simulink model "BANSHEE_GOTO"  (Simulink 8.1)
settings: Solver=ode1  StartTime=0.0  StopTime=inf  FixedStep=Ts  MaxStep=1e-3  RelTol=1e-3
PostLoadFcn:
  | BANSHEE_init;
InitFcn:
  | BANSHEE_init;
values from neighbouring files (symbols this model uses):
  F1 = xlsread('F1_relay_banshee.xlsx')    [relay_settings_init.m]
  F2 = xlsread('F2_relay_banshee.xlsx')    [relay_settings_init.m]
  F3 = xlsread('F3_relay_banshee.xlsx')    [relay_settings_init.m]
  Ts = 100E-6    (= 0.0001)    [BANSHEE_init.m]
undefined symbols (not defined in the file or in its folder): cable_spec, fdesignblkfcn, Feeder1_lib, Feeder2_lib, Feeder3_lib, gcbh, generic_ethernet_cb, Left, relay_housing_lib, SM_UtilityService, SS_F1_RELAY_HOUSING, SS_F2_RELAY_HOUSING, SS_F3_RELAY_HOUSING, SS_Feeder1, SS_Feeder2, SS_Feeder3, type, utility_service_lib, V
libraries: breaker_lib x51, rtio_generic_modbus x43, relay_modbus_lib x42, cables_lib x34, artemis x24, transformer_lib x24, Load_lib x18, simulink x16, ssn_lib x16, rtlab x15, rtio_opalrt_common x15, PQFV_lib x8
(part 2 of 5)

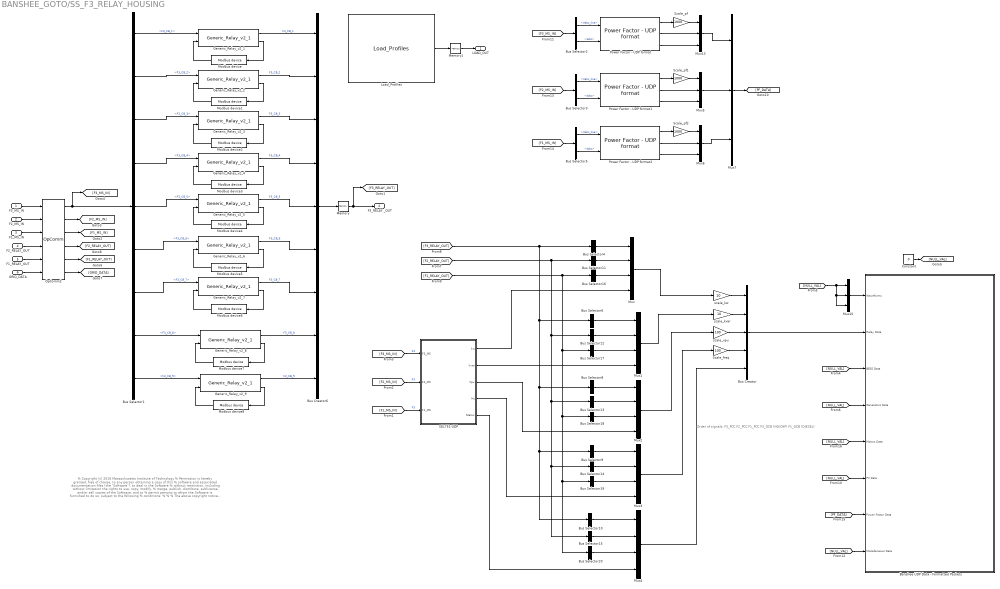
== system BANSHEE_GOTO/SS_F3_RELAY_HOUSING ==
  note: % Copyright (c) 2016 Massachusetts Institute of Technology
      | % Permission is hereby granted, free of charge, to any person obtaining a copy of this
      | % software and associated documentation files (the "Software"), to deal in the Software
      | % without restriction, including without limitation the rights to use, copy, modify,
      | % merge, publish, distribute, sublicense, and/or sell copies of the Software, and to
      | % permit persons to whom the Software is furnished to do so, subject to the following
      | % conditions:
      | %
      | %
      | % The above copyright notice and this permission notice shall be included in
      | % all copies or substantial portions of the Software.
      | %
      | % THE SOFTWARE IS PROVIDED "AS IS", WITHOUT WARRANTY OF ANY KIND, EXPRESS OR IMPLIED,
      | % INCLUDING BUT NOT LIMITED TO THE WARRANTIES OF MERCHANTABILITY, FITNESS FOR A
      | % PARTICULAR PURPOSE AND NONINFRINGEMENT. IN NO EVENT SHALL THE AUTHORS OR COPYRIGHT
      | % HOLDERS BE LIABLE FOR ANY CLAIM, DAMAGES OR OTHER LIABILITY, WHETHER IN AN ACTION
      | % OF CONTRACT, TORT OR OTHERWISE, ARISING FROM, OUT OF OR IN CONNECTION WITH THE
      | % SOFTWARE OR THE USE OR OTHER DEALINGS IN THE SOFTWARE.
      | %
      | %
      | %%
  note: Order of signals:
      | F3_PCC
      | F2_PCC
      | F1_PCC
      | F3_GCB (NG/CHP)
      | F1_GCB (DIESEL)
  F3_MS_IN : Inport
  F2_MS_IN : Inport  Port=2
  F1_MS_IN : Inport  Port=3
  F2_RELAY_OUT : Inport  Port=4
  F1_RELAY_OUT : Inport  Port=5
  GRID_DATA : Inport  Port=6
  Banshee UDP Data - Formatted Packets : Subsystem  mask(UDP Data Block){ProfileID=2, NumOfWaveforms=[0, 0, 0], NumOfRelays=[47, [10, 10, 100, 100]], NumOfBatteries=0, NumOfGensets=0, NumOfMotors=0, NumOfPVs=0, NumOfPF=[3, [1000, 1000, 1000]], NumOfMiscellaneousDataScales=0, NumOfMiscellaneousDataSignalsScales=0}
      mask prompts: ProfileID "Profile ID"; NumOfWaveforms "Waveform Data"; NumOfRelays "Relay Data"; NumOfBatteries "# of Batteries"; NumOfGensets "# of Gensets"; NumOfMotors "# of Motors"; NumOfPVs "# of PVs"; NumOfPF "Power Factor Data"; NumOfMiscellaneousDataScales "Misc. Data - No. of Scale Factors"; NumOfMiscellaneousDataSignalsScales "Misc. - No. Signals and Scale Values"
      mask help:
      | * All signal scaling should be external to this block
      |
      | Profile ID: (1-Sheriff, 2-Banshee, 3-Canary, 4-Siren)
      |
      | Waveforms Data: No. of per phase waveforms sent at 5Hz rate, point per waveforms [dt=80us, 208; dt=100us, 166], and scaling factor.
      | -Input format: [No. of waveforms, No. of datapoints, scale]
      | -Ex. for Canary:[3, 166, 100]
      |
      | Relay Data: No. of relays feeding packet data to breakers in display - mapped/indexed in ascending order
      | -Packet order: Active power(kW), reactive power(kVAR), voltage(per-unit), frequency (Hz), breaker status (1:closed, 0:open)
      | -Input format: [No. of Relays, [scale_kW, scale_kVAR, scale_Vpu, scale_Hz]]
      | -Ex. for Canary:[4, [10, 10, 100, 100]]
      |
      | No. of Batteries: TBD
      | -Ex. for Canary: [0]
      | No. of Generators: TBD
      | -Ex. for Canary: [0]
      |
      | Motors Data: No. of motors monitored in the system. Currently, only looking at motor on/off state.
      | -Input format: [No. of motors]
      | -Ex. for Canary: [1]
      |
      | No. of PV: TBD
      | -Ex. for Canary: [0]
      |
      | Power Factor Data: No. of power factors to be displayed in the system, and corresponding scale values.
      | -Packet order: power factor, import/export, lagging/leading
      | -Input format: [No. of Power Factors, [scale_pf]]
      | -Ex. for Canary:[1, [1000]]
      |
      | Misc. Data - No. of Scale factor: NUmber of scale factors to be applied to each signal-set.
      | -Ex. for Canary: [3]
      |
      | Misc. Data - No. of Signals and Scale Values: Size of signal set and scale value to be applied to the signal-set.
      | -Ex. for Canary: [[1, 1000], [6, 100], [3, 10]]
  Bus Creator : BusCreator  Inputs=5
  Bus Creator6 : BusCreator  Inputs=9
  Bus Selector1 : BusSelector  OutputSignals=CB_DATA.F3_CB_1,CB_DATA.F3_CB_2,CB_DATA.F3_CB_3,CB_DATA.F3_CB_4,CB_DATA.F3_CB_5,CB_DATA.F3_CB_6,CB_DATA.F3_CB_7,CB_DATA.F3_CB_8,CB_DATA.F3_CB_9
  Bus Selector10 : BusSelector  OutputSignals=F3_CB_1.m.status,F3_CB_2.m.status,F3_CB_3.m.status,F3_CB_4.m.status,F3_CB_5.m.status,F3_CB_6.m.status,F3_CB_7.m.status,F3_CB_8.m.status,F3_CB_9.m.status  OutputAsBus=on
  Bus Selector11 : BusSelector  OutputSignals=F2_CB_1.m.kw,F2_CB_2.m.kw,F2_CB_3.m.kw,F2_CB_4.m.kw,F2_CB_5.m.kw,F2_CB_6.m.kw,F2_CB_7.m.kw,F2_CB_8.m.kw,F2_CB_9.m.kw,F2_CB_10.m.kw,F2_CB_11.m.kw,F2_CB_12.m.kw,F2_CB_13.m.kw,F2_CB_14.m.kw,F2_CB_15.m.kw,F2_CB_16.m.kw,F2_CB_17.m.kw,F2_CB_18.m.kw,F2_CB_19.m.kw  OutputAsBus=on
  Bus Selector12 : BusSelector  OutputSignals=F2_CB_1.m.kvar,F2_CB_2.m.kvar,F2_CB_3.m.kvar,F2_CB_4.m.kvar,F2_CB_5.m.kvar,F2_CB_6.m.kvar,F2_CB_7.m.kvar,F2_CB_8.m.kvar,F2_CB_9.m.kvar,F2_CB_10.m.kvar,F2_CB_11.m.kvar,F2_CB_12.m.kvar,F2_CB_13.m.kvar,F2_CB_14.m.kvar,F2_CB_15.m.kvar,F2_CB_16.m.kvar,F2_CB_17.m.kvar,F2_CB_18.m.kvar,F2_CB_19.m.kvar  OutputAsBus=on
  Bus Selector13 : BusSelector  OutputSignals=F2_CB_1.m.Vpu,F2_CB_2.m.Vpu,F2_CB_3.m.Vpu,F2_CB_4.m.Vpu,F2_CB_5.m.Vpu,F2_CB_6.m.Vpu,F2_CB_7.m.Vpu,F2_CB_8.m.Vpu,F2_CB_9.m.Vpu,F2_CB_10.m.Vpu,F2_CB_11.m.Vpu,F2_CB_12.m.Vpu,F2_CB_13.m.Vpu,F2_CB_14.m.Vpu,F2_CB_15.m.Vpu,F2_CB_16.m.Vpu,F2_CB_17.m.Vpu,F2_CB_18.m.Vpu,F2_CB_19.m.Vpu  OutputAsBus=on
  Bus Selector14 : BusSelector  OutputSignals=F2_CB_1.m.Hz,F2_CB_2.m.Hz,F2_CB_3.m.Hz,F2_CB_4.m.Hz,F2_CB_5.m.Hz,F2_CB_6.m.Hz,F2_CB_7.m.Hz,F2_CB_8.m.Hz,F2_CB_9.m.Hz,F2_CB_10.m.Hz,F2_CB_11.m.Hz,F2_CB_12.m.Hz,F2_CB_13.m.Hz,F2_CB_14.m.Hz,F2_CB_15.m.Hz,F2_CB_16.m.Hz,F2_CB_17.m.Hz,F2_CB_18.m.Hz,F2_CB_19.m.Hz  OutputAsBus=on
  Bus Selector15 : BusSelector  OutputSignals=F2_CB_1.m.status,F2_CB_2.m.status,F2_CB_3.m.status,F2_CB_4.m.status,F2_CB_5.m.status,F2_CB_6.m.status,F2_CB_7.m.status,F2_CB_8.m.status,F2_CB_9.m.status,F2_CB_10.m.status,F2_CB_11.m.status,F2_CB_12.m.status,F2_CB_13.m.status,F2_CB_14.m.status,F2_CB_15.m.status,F2_CB_16.m.status,F2_CB_17.m.status,F2_CB_18.m.status,F2_CB_19.m.status  OutputAsBus=on
  Bus Selector16 : BusSelector  OutputSignals=F1_CB_1.m.kw,F1_CB_2.m.kw,F1_CB_3.m.kw,F1_CB_4.m.kw,F1_CB_5.m.kw,F1_CB_6.m.kw,F1_CB_7.m.kw,F1_CB_8.m.kw,F1_CB_9.m.kw,F1_CB_10.m.kw,F1_CB_11.m.kw,F1_CB_12.m.kw,F1_CB_13.m.kw,F1_CB_14.m.kw  OutputAsBus=on
  Bus Selector17 : BusSelector  OutputSignals=F1_CB_1.m.kvar,F1_CB_2.m.kvar,F1_CB_3.m.kvar,F1_CB_4.m.kvar,F1_CB_5.m.kvar,F1_CB_6.m.kvar,F1_CB_7.m.kvar,F1_CB_8.m.kvar,F1_CB_9.m.kvar,F1_CB_10.m.kvar,F1_CB_12.m.kvar,F1_CB_11.m.kvar,F1_CB_13.m.kvar,F1_CB_14.m.kvar  OutputAsBus=on
  Bus Selector18 : BusSelector  OutputSignals=F1_CB_1.m.Vpu,F1_CB_2.m.Vpu,F1_CB_3.m.Vpu,F1_CB_4.m.Vpu,F1_CB_5.m.Vpu,F1_CB_6.m.Vpu,F1_CB_7.m.Vpu,F1_CB_8.m.Vpu,F1_CB_9.m.Vpu,F1_CB_10.m.Vpu,F1_CB_11.m.Vpu,F1_CB_12.m.Vpu,F1_CB_13.m.Vpu,F1_CB_14.m.Vpu  OutputAsBus=on
  Bus Selector19 : BusSelector  OutputSignals=F1_CB_1.m.Hz,F1_CB_2.m.Hz,F1_CB_3.m.Hz,F1_CB_4.m.Hz,F1_CB_5.m.Hz,F1_CB_6.m.Hz,F1_CB_7.m.Hz,F1_CB_8.m.Hz,F1_CB_9.m.Hz,F1_CB_10.m.Hz,F1_CB_11.m.Hz,F1_CB_12.m.Hz,F1_CB_13.m.Hz,F1_CB_14.m.Hz  OutputAsBus=on
  Bus Selector2 : BusSelector  OutputSignals=CB_DATA.F3_PCC.Vabc_line,CB_DATA.F3_PCC.Iabc
  Bus Selector20 : BusSelector  OutputSignals=F1_CB_1.m.status,F1_CB_2.m.status,F1_CB_3.m.status,F1_CB_4.m.status,F1_CB_5.m.status,F1_CB_6.m.status,F1_CB_7.m.status,F1_CB_8.m.status,F1_CB_9.m.status,F1_CB_10.m.status,F1_CB_11.m.status,F1_CB_12.m.status,F1_CB_13.m.status,F1_CB_14.m.status  OutputAsBus=on
  Bus Selector3 : BusSelector  OutputSignals=CB_DATA.F2_PCC.Vabc_line,CB_DATA.F2_PCC.Iabc
  Bus Selector4 : BusSelector  OutputSignals=F3_CB_1.m.kw,F3_CB_2.m.kw,F3_CB_3.m.kw,F3_CB_4.m.kw,F3_CB_5.m.kw,F3_CB_6.m.kw,F3_CB_7.m.kw,F3_CB_8.m.kw,F3_CB_9.m.kw  OutputAsBus=on
  Bus Selector5 : BusSelector  OutputSignals=CB_DATA.F1_PCC.Vabc_line,CB_DATA.F1_PCC.Iabc
  Bus Selector6 : BusSelector  OutputSignals=F3_CB_1.m.kvar,F3_CB_2.m.kvar,F3_CB_3.m.kvar,F3_CB_4.m.kvar,F3_CB_5.m.kvar,F3_CB_6.m.kvar,F3_CB_7.m.kvar,F3_CB_8.m.kvar,F3_CB_9.m.kvar  OutputAsBus=on
  Bus Selector8 : BusSelector  OutputSignals=F3_CB_1.m.Vpu,F3_CB_2.m.Vpu,F3_CB_3.m.Vpu,F3_CB_4.m.Vpu,F3_CB_5.m.Vpu,F3_CB_6.m.Vpu,F3_CB_7.m.Vpu,F3_CB_8.m.Vpu,F3_CB_9.m.Vpu  OutputAsBus=on
  Bus Selector9 : BusSelector  OutputSignals=F3_CB_1.m.Hz,F3_CB_2.m.Hz,F3_CB_3.m.Hz,F3_CB_4.m.Hz,F3_CB_5.m.Hz,F3_CB_6.m.Hz,F3_CB_7.m.Hz,F3_CB_8.m.Hz,F3_CB_9.m.Hz  OutputAsBus=on
  Constant : Constant  Value=0
  Generic_Relay_v2_1 : relay_modbus_lib/Generic_Relay_v2_1  Ts=Ts  relay_settings=[F3(1,:)]
  Generic_Relay_v2_2 : relay_modbus_lib/Generic_Relay_v2_1  Ts=Ts  relay_settings=[F3(2,:)]
  Generic_Relay_v2_3 : relay_modbus_lib/Generic_Relay_v2_1  Ts=Ts  relay_settings=[F3(3,:)]
  Generic_Relay_v2_4 : relay_modbus_lib/Generic_Relay_v2_1  Ts=Ts  relay_settings=[F3(4,:)]
  Generic_Relay_v2_5 : relay_modbus_lib/Generic_Relay_v2_1  Ts=Ts  relay_settings=[F3(5,:)]
  Generic_Relay_v2_6 : relay_modbus_lib/Generic_Relay_v2_1  Ts=Ts  relay_settings=[F3(6,:)]
  Generic_Relay_v2_7 : relay_modbus_lib/Generic_Relay_v2_1  Ts=Ts  relay_settings=[F3(7,:)]
  Generic_Relay_v2_8 : relay_modbus_lib/Generic_Relay_v2_1  Ts=Ts  relay_settings=[F3(8,:)]
  Generic_Relay_v2_9 : relay_modbus_lib/Generic_Relay_v2_1  Ts=Ts  relay_settings=[F3(9,:)]
  Load_Profiles : LoadProfiles_lib/Load_Profiles
  Memory : Memory
  Memory1 : Memory
  Modbus device : rtio_generic_modbus/Modbus device  conf_name=F3_relay_cfg1.opal  conf_name_mask=F3_relay_cfg1.xls  sample_time=Ts
  Modbus device1 : rtio_generic_modbus/Modbus device  conf_name=F3_relay_cfg2.opal  conf_name_mask=F3_relay_cfg2.xls  sample_time=Ts
  Modbus device2 : rtio_generic_modbus/Modbus device  conf_name=F3_relay_cfg3.opal  conf_name_mask=F3_relay_cfg3.xls  sample_time=Ts
  Modbus device3 : rtio_generic_modbus/Modbus device  conf_name=F3_relay_cfg4.opal  conf_name_mask=F3_relay_cfg4.xls  sample_time=Ts
  Modbus device4 : rtio_generic_modbus/Modbus device  conf_name=F3_relay_cfg5.opal  conf_name_mask=F3_relay_cfg5.xls  sample_time=Ts
  Modbus device5 : rtio_generic_modbus/Modbus device  conf_name=F3_relay_cfg6.opal  conf_name_mask=F3_relay_cfg6.xls  sample_time=Ts
  Modbus device6 : rtio_generic_modbus/Modbus device  conf_name=F3_relay_cfg7.opal  conf_name_mask=F3_relay_cfg7.xls  sample_time=Ts
  Modbus device7 : rtio_generic_modbus/Modbus device  conf_name=F3_relay_cfg8.opal  conf_name_mask=F3_relay_cfg8.xls  sample_time=Ts
  Modbus device8 : rtio_generic_modbus/Modbus device  conf_name=F3_relay_cfg9.opal  conf_name_mask=F3_relay_cfg9.xls  sample_time=Ts
  Mux{,1..4} (5 alike) : Mux
  Mux{5..7,10,13} (5 alike) : Mux  Inputs=3
  OpComm2 : rtlab/OpComm  nbport=6  groupe_acq=1  subsys_rate=0  st=0  Synchronization=on  Interpolation=on  Threshold=1.0  Missed_Data=off  Sim_Time=off  Samples=off  dynSigOut=off  from_console=0  warning_done=off  writeOpCommFile=off  Offset=off
  Power Factor - UDP format : udp_powerfactor_lib/Power Factor - UDP format
  Power Factor - UDP format1 : udp_powerfactor_lib/Power Factor - UDP format
  Power Factor - UDP format2 : udp_powerfactor_lib/Power Factor - UDP format
  SEL751-UDP : Subsystem
  Scale_freq : Gain  Gain=100
  Scale_pf : Gain  Gain=1000
  Scale_pf1 : Gain  Gain=1000
  Scale_pf2 : Gain  Gain=1000
  scale_kvar : Gain  Gain=10
  scale_kw : Gain  Gain=10
  scale_vpu : Gain  Gain=100
  LOAD_OUT : Outport
  F3_RELAY _OUT : Outport  Port=2
  wires:
  Load_Profiles/1 -> Memory1/1
  OpComm2/1 -> Bus Selector1/1, [F3_MS_IN]
  Generic_Relay_v2_1/2 -> Modbus device/1
  Modbus device/1 -> Generic_Relay_v2_1/2
  Generic_Relay_v2_2/2 -> Modbus device1/1
  Modbus device1/1 -> Generic_Relay_v2_2/2
  Modbus device2/1 -> Generic_Relay_v2_3/2
  Generic_Relay_v2_3/2 -> Modbus device2/1
  Generic_Relay_v2_4/2 -> Modbus device3/1
  Modbus device3/1 -> Generic_Relay_v2_4/2
  Generic_Relay_v2_5/2 -> Modbus device4/1
  Modbus device4/1 -> Generic_Relay_v2_5/2
  Modbus device5/1 -> Generic_Relay_v2_6/2
  Generic_Relay_v2_6/2 -> Modbus device5/1
  Generic_Relay_v2_7/2 -> Modbus device6/1
  Modbus device6/1 -> Generic_Relay_v2_7/2
  F3_MS_IN/1 -> OpComm2/1
  Bus Selector1/1 -> Generic_Relay_v2_1/1  "<F3_CB_1>"
  Bus Selector1/2 -> Generic_Relay_v2_2/1  "<F3_CB_2>"
  Bus Selector1/3 -> Generic_Relay_v2_3/1  "<F3_CB_3>"
  Bus Selector1/4 -> Generic_Relay_v2_4/1  "<F3_CB_4>"
  Bus Selector1/5 -> Generic_Relay_v2_5/1  "<F3_CB_5>"
  Bus Selector1/6 -> Generic_Relay_v2_6/1  "<F3_CB_6>"
  Bus Selector1/7 -> Generic_Relay_v2_7/1  "<F3_CB_7>"
  Generic_Relay_v2_1/1 -> Bus Creator6/1  "F3_CB_1"
  Generic_Relay_v2_2/1 -> Bus Creator6/2  "F3_CB_2"
  Generic_Relay_v2_3/1 -> Bus Creator6/3  "F3_CB_3"
  Generic_Relay_v2_4/1 -> Bus Creator6/4  "F3_CB_4"
  Generic_Relay_v2_5/1 -> Bus Creator6/5  "F3_CB_5"
  Generic_Relay_v2_6/1 -> Bus Creator6/6  "F3_CB_6"
  Generic_Relay_v2_7/1 -> Bus Creator6/7  "F3_CB_7"
  Bus Creator6/1 -> Memory/1
  Modbus device7/1 -> Generic_Relay_v2_8/2
  Generic_Relay_v2_8/2 -> Modbus device7/1
  Generic_Relay_v2_9/2 -> Modbus device8/1
  Modbus device8/1 -> Generic_Relay_v2_9/2
  Generic_Relay_v2_8/1 -> Bus Creator6/8  "F3_CB_8"
  Generic_Relay_v2_9/1 -> Bus Creator6/9  "F3_CB_9"
  Bus Selector1/9 -> Generic_Relay_v2_9/1  "<F3_CB_9>"
  Bus Selector1/8 -> Generic_Relay_v2_8/1  "<F3_CB_8>"
  Memory/1 -> [F3_RELAY_OUT], F3_RELAY _OUT/1
  Memory1/1 -> LOAD_OUT/1
  F2_RELAY_OUT/1 -> OpComm2/4
  F1_RELAY_OUT/1 -> OpComm2/5
  OpComm2/4 -> [F2_RELAY_OUT]
  OpComm2/5 -> [F1_RELAY_OUT]
  OpComm2/2 -> [F2_MS_IN]
  OpComm2/3 -> [F1_MS_IN]
  F2_MS_IN/1 -> OpComm2/2
  F1_MS_IN/1 -> OpComm2/3
  [F3_MS_IN] -> SEL751-UDP/1(F3_MS)  "F3"
  [F2_MS_IN] -> SEL751-UDP/2(F2_MS)  "F3"
  [F1_MS_IN] -> SEL751-UDP/3(F1_MS)  "F3"
  [NULL_VAL] -> Mux10/3, Mux10/2, Mux10/1
  Mux10/1 -> Banshee UDP Data - Formatted Packets/1(Waveforms)
  Constant/1 -> [NULL_VAL]
  Bus Creator/1 -> Banshee UDP Data - Formatted Packets/2(Relay Data)
  scale_kw/1 -> Bus Creator/1
  scale_kvar/1 -> Bus Creator/2
  Scale_freq/1 -> Bus Creator/4
  scale_vpu/1 -> Bus Creator/3
  Mux/1 -> scale_kw/1
  Mux1/1 -> scale_kvar/1
  Mux2/1 -> scale_vpu/1
  Mux3/1 -> Scale_freq/1
  Mux4/1 -> Bus Creator/5
  [NULL_VAL] -> Banshee UDP Data - Formatted Packets/4(Generators Data)
  [NULL_VAL] -> Banshee UDP Data - Formatted Packets/3(BESS Data)
  [NULL_VAL] -> Banshee UDP Data - Formatted Packets/5(Motors Data)
  [NULL_VAL] -> Banshee UDP Data - Formatted Packets/6(PV Data)
  Power Factor - UDP format/1 -> Scale_pf/1
  Scale_pf/1 -> Mux13/1
  [F3_MS_IN] -> Bus Selector2/1
  Bus Selector2/1 -> Power Factor - UDP format/1  "<Vabc_line>"
  Bus Selector2/2 -> Power Factor - UDP format/2  "<Iabc>"
  Power Factor - UDP format/2 -> Mux13/2
  Power Factor - UDP format/3 -> Mux13/3
  Mux13/1 -> Mux7/1
  [NULL_VAL] -> Banshee UDP Data - Formatted Packets/8(Miscellaneous Data)
  Power Factor - UDP format1/1 -> Scale_pf1/1
  Scale_pf1/1 -> Mux5/1
  [F2_MS_IN] -> Bus Selector3/1
  Bus Selector3/1 -> Power Factor - UDP format1/1  "<Vabc_line>"
  Bus Selector3/2 -> Power Factor - UDP format1/2  "<Iabc>"
  Power Factor - UDP format1/2 -> Mux5/2
  Power Factor - UDP format1/3 -> Mux5/3
  Mux5/1 -> Mux7/2
  Power Factor - UDP format2/1 -> Scale_pf2/1
  Scale_pf2/1 -> Mux6/1
  [F1_MS_IN] -> Bus Selector5/1
  Bus Selector5/1 -> Power Factor - UDP format2/1  "<Vabc_line>"
  Bus Selector5/2 -> Power Factor - UDP format2/2  "<Iabc>"
  Power Factor - UDP format2/2 -> Mux6/2
  Power Factor - UDP format2/3 -> Mux6/3
  Mux6/1 -> Mux7/3
  Mux7/1 -> [PF_DATA]
  [PF_DATA] -> Banshee UDP Data - Formatted Packets/7(Power Factor Data)
  OpComm2/6 -> [GRID_DATA]
  GRID_DATA/1 -> OpComm2/6
  Bus Selector4/1 -> Mux/1
  Bus Selector6/1 -> Mux1/1
  Bus Selector8/1 -> Mux2/1
  Bus Selector9/1 -> Mux3/1
  Bus Selector10/1 -> Mux4/1
  [F3_RELAY_OUT] -> Bus Selector10/1, Bus Selector9/1, Bus Selector8/1, Bus Selector6/1, Bus Selector4/1
  Bus Selector12/1 -> Mux1/2
  Bus Selector11/1 -> Mux/2
  Bus Selector13/1 -> Mux2/2
  Bus Selector15/1 -> Mux4/2
  Bus Selector14/1 -> Mux3/2
  [F2_RELAY_OUT] -> Bus Selector15/1, Bus Selector14/1, Bus Selector13/1, Bus Selector12/1, Bus Selector11/1
  Bus Selector20/1 -> Mux4/3
  Bus Selector19/1 -> Mux3/3
  Bus Selector18/1 -> Mux2/3
  Bus Selector17/1 -> Mux1/3
  Bus Selector16/1 -> Mux/3
  [F1_RELAY_OUT] -> Bus Selector17/1, Bus Selector18/1, Bus Selector20/1, Bus Selector19/1, Bus Selector16/1
  SEL751-UDP/1(kw) -> Mux/4
  SEL751-UDP/2(kvar) -> Mux1/4
  SEL751-UDP/3(Vpu) -> Mux2/4
  SEL751-UDP/4(Hz) -> Mux3/4
  SEL751-UDP/5(Status) -> Mux4/4

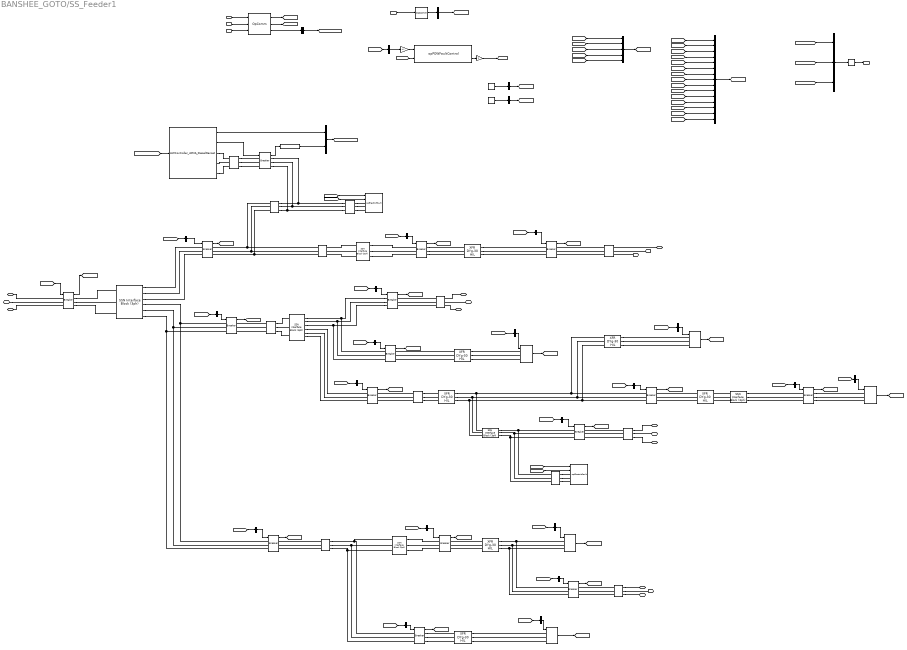
== system BANSHEE_GOTO/SS_Feeder1 ==
  note: motor
  note: connect to F2
  note: connect to F2
  note: connect to F2
  note: connect to F3
  note: % Copyright (c) 2016 Massachusetts Institute of Technology
      | % Permission is hereby granted, free of charge, to any person obtaining a copy of this
      | % software and associated documentation files (the "Software"), to deal in the Software
      | % without restriction, including without limitation the rights to use, copy, modify,
      | % merge, publish, distribute, sublicense, and/or sell copies of the Software, and to
      | % permit persons to whom the Software is furnished to do so, subject to the following
      | % conditions:
      | %
      | %
      | % The above copyright notice and this permission notice shall be included in
      | % all copies or substantial portions of the Software.
      | %
      | % THE SOFTWARE IS PROVIDED "AS IS", WITHOUT WARRANTY OF ANY KIND, EXPRESS OR IMPLIED,
      | % INCLUDING BUT NOT LIMITED TO THE WARRANTIES OF MERCHANTABILITY, FITNESS FOR A
      | % PARTICULAR PURPOSE AND NONINFRINGEMENT. IN NO EVENT SHALL THE AUTHORS OR COPYRIGHT
      | % HOLDERS BE LIABLE FOR ANY CLAIM, DAMAGES OR OTHER LIABILITY, WHETHER IN AN ACTION
      | % OF CONTRACT, TORT OR OTHERWISE, ARISING FROM, OUT OF OR IN CONNECTION WITH THE
      | % SOFTWARE OR THE USE OR OTHER DEALINGS IN THE SOFTWARE.
      | %
      | %
      | %%
  note: Point-on-wave synchronisation voltage (3-phase) in PU - Using 13.8 kV
  RELAY_IN : Inport
  LOAD_IN : Inport  Port=2
  SC_CMD : Inport  Port=3
  HWCtrl_CMD : Inport  Port=4
  2000 kVA4 : transformer_lib/XFR DYg-30 HIL  Rating=2000  Vp=4160  Vs=480  Z=5.75  XR=5.7
  2000 kVA5 : transformer_lib/XFR DYg-30 HIL  Rating=2000  Vp=4160  Vs=480  Z=5.75  XR=5.7
  2500 kVA : transformer_lib/XFR DYg-30 HIL  Rating=2500  Vp=13800  Vs=480  Z=5.75  XR=6.6
  2500 kVA2 : transformer_lib/XFR DYg-30 HIL  Rating=2500  Vp=13800  Vs=480  Z=5.56  XR=5.52
  3750 kVA1 : transformer_lib/XFR DYg-30 HIL  Rating=3750  Vp=13800  Vs=4160  Z=4.75  XR=11.4
  500 kVA2 : transformer_lib/XFR DYg-30 HIL  Rating=500  Vp=13800  Vs=480  Z=5  XR=4.9
  500 kVA3 : transformer_lib/XFR DYg-30 HIL  Rating=500  Vp=13800  Vs=208  Z=5  XR=4.9
  500kcmil_cable : cables_lib/500kcmil_cable  length=1  par_sets=1
  500kcmil_cable1 : cables_lib/500kcmil_cable  length=1  par_sets=1
  Bus Creator : BusCreator  Inputs=1
  Bus Creator1 : BusCreator  Inputs=1
  Bus Creator2 : BusCreator  Inputs=3
  Bus Creator3 : BusCreator  Inputs=5
  Bus Creator5 : BusCreator  Inputs=15
  Bus Creator6 : BusCreator  Inputs=2
  Bus Selector : BusSelector  OutputSignals=Vabc_bus
  Bus Selector1 : BusSelector  OutputSignals=F1_CB_12
  Bus Selector10 : BusSelector  OutputSignals=F1_CB_2
  Bus Selector11 : BusSelector  OutputSignals=F1_CB_1
  Bus Selector12 : BusSelector  OutputSignals=F1_CB_5
  Bus Selector13 : BusSelector  OutputSignals=F1_CB_3
  Bus Selector14 : BusSelector  OutputSignals=F1_CB_6
  Bus Selector15 : BusSelector  OutputSignals=F1_CB_7
  Bus Selector16 : BusSelector  OutputSignals=F1_CB_10
  Bus Selector17 : BusSelector  OutputSignals=F1_CB_11
  Bus Selector18 : BusSelector  OutputSignals=F1_CB_9
  Bus Selector19 : BusSelector  OutputSignals=F1_CB_14
  Bus Selector2 : BusSelector  OutputSignals=F1_CB_4
  Bus Selector20 : BusSelector  OutputSignals=fault_cmd
  Bus Selector21 : BusSelector  OutputSignals=Diesel_Gen2
  Bus Selector3 : BusSelector  OutputSignals=I2
  Bus Selector4 : BusSelector  OutputSignals=C2
  Bus Selector5 : BusSelector  OutputSignals=P1
  Bus Selector6 : BusSelector  OutputSignals=C1
  Bus Selector7 : BusSelector  OutputSignals=I1
  Bus Selector8 : BusSelector  OutputSignals=F1_CB_13
  Bus Selector9 : BusSelector  OutputSignals=F1_CB_8
  C101 : cables_lib/PI-Section  cable_spec=[cable_spec(13, :)]  line_length=1800  parallel_sets=1
  C102 : cables_lib/PI-Section  cable_spec=[cable_spec(13, :)]  line_length=5500  parallel_sets=1
  C103 : cables_lib/PI-Section  cable_spec=[cable_spec(11, :)]  line_length=1000  parallel_sets=1
  C104 : cables_lib/PI-Section  cable_spec=[cable_spec(13, :)]  line_length=3000  parallel_sets=1
  C105 : cables_lib/PI-Section  cable_spec=[cable_spec(13, :)]  line_length=3000  parallel_sets=1
  C106 : cables_lib/PI-Section  cable_spec=[cable_spec(13, :)]  line_length=1500  parallel_sets=1
  C107 : cables_lib/PI-Section  cable_spec=[cable_spec(6, :)]  line_length=2000  parallel_sets=2
  C108 : cables_lib/PI-Section  cable_spec=[cable_spec(6, :)]  line_length=1000  parallel_sets=2
  C109 : cables_lib/PI-Section  cable_spec=[cable_spec(6, :)]  line_length=2000  parallel_sets=2
  CB closed : Constant
  CB open : Constant  Value=0
  Critical_1 : Load_lib/Dynamic_Load  V=460  Ts=Ts
  Critical_2 : Load_lib/Dynamic_Load  V=460  Ts=Ts
  F1-GCB : breaker_lib/Breaker  Ts=Ts  mech_delay=cb_mech_delay
  F1_CB_{1..14} (14 alike) : breaker_lib/Breaker  Ts=Ts  mech_delay=cb_mech_delay
  F1_PCC : breaker_lib/Breaker  Ts=Ts  mech_delay=cb_mech_delay
  HWController_4MVA_DieselGenset : HWController_Diesel_GenSet_4MVA_lib/HWController_4MVA_DieselGenset
  Interruptible_1 : Load_lib/Dynamic_Load  V=460  Ts=Ts
  Interruptible_2 : Load_lib/Dynamic_Load  V=208  Ts=Ts
  Memory : Memory
  OpComm1 : rtlab/OpComm  nbport=3  groupe_acq=1  subsys_rate=0  st=0  Synchronization=on  Interpolation=on  Threshold=1.0  Missed_Data=off  Sim_Time=off  Samples=off  dynSigOut=off  from_console=0  warning_done=off  writeOpCommFile=off  Offset=off
  OpComm2 : rtlab/OpComm  nbport=1  groupe_acq=1  subsys_rate=0  st=0  Synchronization=on  Interpolation=on  Threshold=1.0  Missed_Data=off  Sim_Time=off  Samples=off  dynSigOut=off  from_console=1  warning_done=off  writeOpCommFile=off  Offset=off
  PI-Section4 : cables_lib/PI-Section  cable_spec=[cable_spec(11, :)]  line_length=2000  parallel_sets=1
  PQFV : PQFV_lib/PQFV  VRMSLL=13800
  Priority_1 : Load_lib/Dynamic_Load  V=460  Ts=Ts
  SSN Interface Block (3ph) : ssn_lib/SSN Interface Block (3ph)  nb_phase=3  nb_port=3  p1_type=V-type(Left)  p2_type=V-type (Right)  p3_type=V-type (Right)  p4_type=V-type (Right)  p5_type=V-type(Left)  p6_type=V-type(Left)  p7_type=V-type(Left)  p8_type=V-type(Left)  p9_type=V-type(Left)  p10_type=V-type(Left)  p11_type=V-type(Left)  p12_type=V-type(Left)  p13_type=V-type(Left)  p14_type=V-type(Left)  p15_type=V-type(Left)  p16_type=V-type(Left)  I_port_shunt_resistance=1e9
  SSN Interface Block (3ph)1 : ssn_lib/SSN Interface Block (3ph)  nb_phase=3  nb_port=3  p1_type=V-type(Left)  p2_type=V-type (Right)  p3_type=V-type (Right)  p4_type=V-type(Left)  p5_type=V-type(Left)  p6_type=V-type(Left)  p7_type=V-type(Left)  p8_type=V-type(Left)  p9_type=V-type(Left)  p10_type=V-type(Left)  p11_type=V-type(Left)  p12_type=V-type(Left)  p13_type=V-type(Left)  p14_type=V-type(Left)  p15_type=V-type(Left)  p16_type=V-type(Left)  I_port_shunt_resistance=1e9
  SSN Interface Block (3ph){2..4,12} (4 alike) : ssn_lib/SSN Interface Block (3ph)  nb_phase=3  nb_port=2  p1_type=V-type(Left)  p2_type=V-type (Right)  p3_type=V-type(Left)  p4_type=V-type(Left)  p5_type=V-type(Left)  p6_type=V-type(Left)  p7_type=V-type(Left)  p8_type=V-type(Left)  p9_type=V-type(Left)  p10_type=V-type(Left)  p11_type=V-type(Left)  p12_type=V-type(Left)  p13_type=V-type(Left)  p14_type=V-type(Left)  p15_type=V-type(Left)  p16_type=V-type(Left)  I_port_shunt_resistance=1e9
  a : Gain  Gain=1/(13800*sqrt(2/3))
  opElectricFault : artemis/Tools /POW faults/opElectricFault  FaultLocation=location 2  FaultResistance=0.0001  GroundResistance=0.0001  InitialStates=[0 0 0]  SnubberResistance=1e6  SnubberCapacitance=inf
  opElectricFault1 : artemis/Tools /POW faults/opElectricFault  FaultLocation=location 3  FaultResistance=0.0001  GroundResistance=0.0001  InitialStates=[0 0 0]  SnubberResistance=1e6  SnubberCapacitance=inf
  opPOWFaultControl1 : artemis/Tools /POW faults/opPOWFaultControl  Ts=Ts  usePLL=off  Fgrid=60  PLL_k=[180 3200 1]  vol_sel=1: rising zero-corssing  SyncPhase_menu=A  T_acq=0.8
  triggerFAULT : Gain
  A_PCC : PMIOPort  Port=1  Side=Left
  B_PCC : PMIOPort  Port=2  Side=Left
  C_PCC : PMIOPort  Port=3  Side=Left
  A_CB_8 : PMIOPort  Port=4  Side=Right
  B_CB_8 : PMIOPort  Port=5  Side=Right
  C_CB_8 : PMIOPort  Port=6  Side=Right
  A_CB_11 : PMIOPort  Port=7  Side=Right
  B_CB_11 : PMIOPort  Port=8  Side=Right
  C_CB_11 : PMIOPort  Port=9  Side=Right
  A_CB_9 : PMIOPort  Port=10  Side=Right
  B_CB_9 : PMIOPort  Port=11  Side=Right
  C_CB_9 : PMIOPort  Port=12  Side=Right
  A_CB_13 : PMIOPort  Port=13  Side=Right
  B_CB_13 : PMIOPort  Port=14  Side=Right
  C_CB_13 : PMIOPort  Port=15  Side=Right
  DATA_OUT : Outport
  wires:
  [cb_c] -> F1_PCC/1
  F1_PCC/1 -> [F1_PCC]
  Bus Creator/1 -> [cb_c]
  CB closed/1 -> Bus Creator/1  "Logic_trip"
  Bus Creator1/1 -> [cb_o]
  CB open/1 -> Bus Creator1/1  "Logic_trip"
  LOAD_IN/1 -> OpComm1/1
  OpComm1/1 -> [LOAD_IN]
  [LOAD_IN] -> Bus Selector3/1
  [LOAD_IN] -> Bus Selector4/1
  [LOAD_IN] -> Bus Selector5/1
  [LOAD_IN] -> Bus Selector6/1
  [LOAD_IN] -> Bus Selector7/1
  Bus Selector3/1 -> Interruptible_2/1  "<I2>"
  Bus Selector4/1 -> Critical_2/1  "<C2>"
  Bus Selector5/1 -> Priority_1/1  "<P1>"
  Bus Selector6/1 -> Critical_1/1  "<C1>"
  Bus Selector7/1 -> Interruptible_1/1  "<I1>"
  Interruptible_2/1 -> [LOAD_I2]
  Critical_2/1 -> [LOAD_C2]
  Priority_1/1 -> [LOAD_P1]
  Critical_1/1 -> [LOAD_C1]
  Interruptible_1/1 -> [LOAD_I1]
  [LOAD_C1] -> Bus Creator3/1  "F1_C1"
  [LOAD_I2] -> Bus Creator3/4  "F1_I2"
  [LOAD_P1] -> Bus Creator3/5  "F1_P1"
  [LOAD_C2] -> Bus Creator3/2  "F1_C2"
  [LOAD_I1] -> Bus Creator3/3  "F1_I1"
  F1_CB_3/1 -> [F1_CB_3]
  F1_CB_1/1 -> [F1_CB_1]
  F1_CB_5/1 -> [F1_CB_5]
  F1_CB_9/1 -> [F1_CB_9]
  F1_CB_6/1 -> [F1_CB_6]
  F1_CB_7/1 -> [F1_CB_7]
  F1_CB_8/1 -> [F1_CB_8]
  F1_CB_12/1 -> [F1_CB_12]
  F1_CB_13/1 -> [F1_CB_13]
  F1_CB_10/1 -> [F1_CB_10]
  F1_CB_11/1 -> [F1_CB_11]
  [F1_CB_1] -> Bus Creator5/1  "F1_CB_1"
  [F1_CB_13] -> Bus Creator5/13  "F1_CB_13"
  [F1_CB_12] -> Bus Creator5/12  "F1_CB_12"
  [F1_CB_11] -> Bus Creator5/11  "F1_CB_11"
  [F1_CB_10] -> Bus Creator5/10  "F1_CB_10"
  [F1_CB_9] -> Bus Creator5/9  "F1_CB_9"
  [F1_CB_8] -> Bus Creator5/8  "F1_CB_8"
  [F1_CB_7] -> Bus Creator5/7  "F1_CB_7"
  [F1_CB_6] -> Bus Creator5/6  "F1_CB_6"
  [F1_CB_5] -> Bus Creator5/5  "F1_CB_5"
  [F1_CB_4] -> Bus Creator5/4  "F1_CB_4"
  [F1_CB_3] -> Bus Creator5/3  "F1_CB_3"
  [F1_CB_2] -> Bus Creator5/2  "F1_CB_2"
  RELAY_IN/1 -> OpComm1/2
  OpComm1/2 -> [RELAY_IN]
  Bus Selector13/1 -> F1_CB_3/1  "<F1_CB_3>"
  [RELAY_IN] -> Bus Selector13/1
  [RELAY_IN] -> Bus Selector1/1
  [RELAY_IN] -> Bus Selector8/1
  [RELAY_IN] -> Bus Selector9/1
  [RELAY_IN] -> Bus Selector10/1
  [RELAY_IN] -> Bus Selector11/1
  [RELAY_IN] -> Bus Selector12/1
  [RELAY_IN] -> Bus Selector14/1
  [RELAY_IN] -> Bus Selector15/1
  [RELAY_IN] -> Bus Selector16/1
  [RELAY_IN] -> Bus Selector17/1
  [RELAY_IN] -> Bus Selector18/1
  Bus Selector1/1 -> F1_CB_12/1  "<F1_CB_12>"
  Bus Selector8/1 -> F1_CB_13/1  "<F1_CB_13>"
  Bus Selector9/1 -> F1_CB_8/1  "<F1_CB_8>"
  Bus Selector15/1 -> F1_CB_7/1  "<F1_CB_7>"
  Bus Selector14/1 -> F1_CB_6/1  "<F1_CB_6>"
  Bus Selector10/1 -> F1_CB_2/1  "<F1_CB_2>"
  Bus Selector16/1 -> F1_CB_10/1  "<F1_CB_10>"
  Bus Selector17/1 -> F1_CB_11/1  "<F1_CB_11>"
  Bus Selector11/1 -> F1_CB_1/1  "<F1_CB_1>"
  Bus Selector12/1 -> F1_CB_5/1  "<F1_CB_5>"
  Bus Selector18/1 -> F1_CB_9/1  "<F1_CB_9>"
  F1_CB_2/1 -> [F1_CB_2]
  F1_CB_4/1 -> [F1_CB_4]
  [RELAY_IN] -> Bus Selector2/1
  Bus Selector2/1 -> F1_CB_4/1  "<F1_CB_4>"
  F1_CB_14/1 -> [F1_CB_14]
  [RELAY_IN] -> Bus Selector19/1
  Bus Selector19/1 -> F1_CB_14/1  "<F1_CB_14>"
  [F1_PCC] -> Bus Creator5/15  "F1_PCC"
  [F1_CB_14] -> Bus Creator5/14  "F1_CB_14"
  [fault_cmd] -> opPOWFaultControl1/2
  opPOWFaultControl1/2 -> triggerFAULT/1
  triggerFAULT/1 -> [trigger]  "triggerFAULTsig"
  [F1_PCC] -> Bus Selector/1
  Bus Selector/1 -> a/1  "<Vabc_bus>"
  a/1 -> opPOWFaultControl1/1
  SC_CMD/1 -> OpComm2/1
  [fault_cmd] -> opElectricFault/2
  [trigger] -> opElectricFault/1
  [fault_cmd] -> opElectricFault1/2
  [trigger] -> opElectricFault1/1
  OpComm2/1 -> Bus Selector20/1
  Bus Selector20/1 -> [fault_cmd]  "<fault_cmd>"
  Bus Creator3/1 -> [LOAD_DATA]  "LOAD"
  Bus Creator5/1 -> [CB_DATA]
  [Diesel_Gen2] -> HWController_4MVA_DieselGenset/1
  HWController_4MVA_DieselGenset/2 -> F1-GCB/1
  OpComm1/3 -> Bus Selector21/1
  Bus Selector21/1 -> [Diesel_Gen2]  "<Diesel_Gen2>"
  HWCtrl_CMD/1 -> OpComm1/3
  F1-GCB/1 -> PQFV/1
  Bus Creator6/1 -> [DIESEL_DATA]
  PQFV/1 -> Bus Creator6/2  "DIESEL_GCB"
  HWController_4MVA_DieselGenset/1 -> Bus Creator6/1  "Gen2_meas"
  Memory/1 -> DATA_OUT/1
  Bus Creator2/1 -> Memory/1
  [CB_DATA] -> Bus Creator2/1  "CB_DATA"
  [LOAD_DATA] -> Bus Creator2/2  "LOAD_DATA"
  [DIESEL_DATA] -> Bus Creator2/3  "DIESEL_DATA"
  connections:
  C107/LConn3 -- F1_CB_11/RConn3
  C107/LConn2 -- F1_CB_11/RConn2
  C107/LConn1 -- F1_CB_11/RConn1
  C102/RConn1 -- SSN Interface Block (3ph)1/LConn1
  C102/RConn3 -- SSN Interface Block (3ph)1/LConn3
  C102/RConn2 -- SSN Interface Block (3ph)1/LConn2
  2500 kVA2/RConn2 -- Critical_1/LConn2 -- F1_CB_9/LConn2
  C106/LConn1 -- F1_CB_6/RConn1
  2500 kVA/RConn2 -- F1_CB_13/LConn2
  2500 kVA2/LConn3 -- F1_CB_5/RConn3
  C102/LConn2 -- F1_CB_2/RConn2
  2500 kVA2/LConn2 -- F1_CB_5/RConn2
  C102/LConn3 -- F1_CB_2/RConn3
  C102/LConn1 -- F1_CB_2/RConn1
  2500 kVA2/RConn1 -- Critical_1/LConn1 -- F1_CB_9/LConn1
  F1_CB_4/LConn3 -- C101/RConn3 -- SSN Interface Block (3ph)2/LConn3
  F1_CB_12/RConn1 -- 2500 kVA/LConn1
  F1_CB_1/LConn3 -- F1_CB_2/LConn3 -- SSN Interface Block (3ph)/RConn6
  F1_CB_1/LConn2 -- F1_CB_2/LConn2 -- SSN Interface Block (3ph)/RConn5
  F1_CB_1/LConn1 -- F1_CB_2/LConn1 -- SSN Interface Block (3ph)/RConn4
  C106/LConn2 -- F1_CB_6/RConn2
  A_PCC/RConn1 -- F1_PCC/LConn1
  2000 kVA5/LConn1 -- F1_CB_10/RConn1
  2500 kVA2/LConn1 -- F1_CB_5/RConn1
  B_PCC/RConn1 -- F1_PCC/LConn2
  C104/LConn2 -- C103/LConn2 -- F1_CB_3/RConn2
  C106/LConn3 -- F1_CB_6/RConn3
  2000 kVA5/LConn2 -- F1_CB_10/RConn2
  F1_CB_12/RConn2 -- 2500 kVA/LConn2
  C101/LConn1 -- F1_CB_1/RConn1
  F1_CB_12/RConn3 -- 2500 kVA/LConn3
  500 kVA3/LConn3 -- F1_CB_7/RConn3
  C101/LConn2 -- F1_CB_1/RConn2
  2000 kVA5/LConn3 -- F1_CB_10/RConn3
  C104/LConn1 -- C103/LConn1 -- F1_CB_3/RConn1
  C108/LConn1 -- F1_CB_9/RConn1
  C108/LConn2 -- F1_CB_9/RConn2
  C101/LConn3 -- F1_CB_1/RConn3
  C104/LConn3 -- C103/LConn3 -- F1_CB_3/RConn3
  C108/LConn3 -- F1_CB_9/RConn3
  2500 kVA/RConn1 -- F1_CB_13/LConn1
  500 kVA3/LConn1 -- F1_CB_7/RConn1
  500 kVA3/LConn2 -- F1_CB_7/RConn2
  F1_CB_4/LConn2 -- C101/RConn2 -- SSN Interface Block (3ph)2/LConn2
  C_PCC/RConn1 -- F1_PCC/LConn3
  2500 kVA/RConn3 -- F1_CB_13/LConn3
  F1_CB_4/LConn1 -- C101/RConn1 -- SSN Interface Block (3ph)2/LConn1
  2500 kVA2/RConn3 -- Critical_1/LConn3 -- F1_CB_9/LConn3
  500kcmil_cable1/LConn3 -- SSN Interface Block (3ph)12/RConn3 -- F1_CB_11/LConn3
  2000 kVA4/LConn2 -- F1_CB_10/LConn2 -- SSN Interface Block (3ph)12/LConn2 -- 3750 kVA1/RConn2
  500kcmil_cable1/LConn1 -- F1_CB_11/LConn1 -- SSN Interface Block (3ph)12/RConn1
  C108/RConn3 -- C_CB_9/RConn1
  C108/RConn1 -- A_CB_9/RConn1
  C108/RConn2 -- B_CB_9/RConn1
  C107/RConn1 -- A_CB_11/RConn1
  C107/RConn3 -- C_CB_11/RConn1
  C107/RConn2 -- B_CB_11/RConn1
  F1_CB_4/RConn1 -- 500 kVA2/LConn1
  F1_CB_4/RConn3 -- 500 kVA2/LConn3
  F1_CB_4/RConn2 -- 500 kVA2/LConn2
  F1_CB_14/RConn1 -- Priority_1/LConn1
  F1_CB_14/RConn2 -- Priority_1/LConn2
  F1_CB_14/RConn3 -- Priority_1/LConn3
  SSN Interface Block (3ph)2/RConn2 -- F1_CB_5/LConn2
  SSN Interface Block (3ph)2/RConn1 -- F1_CB_5/LConn1
  SSN Interface Block (3ph)2/RConn3 -- F1_CB_5/LConn3
  SSN Interface Block (3ph)/RConn1 -- F1_CB_3/LConn1
  SSN Interface Block (3ph)/RConn2 -- F1_CB_3/LConn2
  SSN Interface Block (3ph)/RConn3 -- F1_CB_3/LConn3
  F1_PCC/RConn2 -- SSN Interface Block (3ph)/LConn2
  F1_PCC/RConn1 -- SSN Interface Block (3ph)/LConn1
  F1_PCC/RConn3 -- SSN Interface Block (3ph)/LConn3
  C109/LConn1 -- F1_CB_13/RConn1
  C109/LConn3 -- F1_CB_13/RConn3
  C109/LConn2 -- F1_CB_13/RConn2
  C_CB_13/RConn1 -- C109/RConn3
  B_CB_13/RConn1 -- C109/RConn2
  A_CB_13/RConn1 -- C109/RConn1
  C105/LConn2 -- F1_CB_8/RConn2
  C105/LConn3 -- F1_CB_8/RConn3
  C105/LConn1 -- F1_CB_8/RConn1
  A_CB_8/RConn1 -- C105/RConn1
  C_CB_8/RConn1 -- C105/RConn3
  B_CB_8/RConn1 -- C105/RConn2
  SSN Interface Block (3ph)3/LConn2 -- C104/RConn2
  SSN Interface Block (3ph)3/LConn3 -- C104/RConn3
  SSN Interface Block (3ph)3/LConn1 -- C104/RConn1
  SSN Interface Block (3ph)3/RConn2 -- F1_CB_12/LConn2
  SSN Interface Block (3ph)3/RConn1 -- F1_CB_12/LConn1
  SSN Interface Block (3ph)3/RConn3 -- F1_CB_12/LConn3
  2000 kVA4/LConn3 -- SSN Interface Block (3ph)12/LConn3 -- 3750 kVA1/RConn3 -- F1_CB_10/LConn3
  500kcmil_cable1/LConn2 -- SSN Interface Block (3ph)12/RConn2 -- F1_CB_11/LConn2
  F1_CB_10/LConn1 -- SSN Interface Block (3ph)12/LConn1 -- 3750 kVA1/RConn1 -- 2000 kVA4/LConn1
  F1_CB_8/LConn1 -- SSN Interface Block (3ph)1/RConn1 -- F1_CB_7/LConn1
  F1_CB_8/LConn2 -- SSN Interface Block (3ph)1/RConn2 -- F1_CB_7/LConn2
  F1_CB_8/LConn3 -- SSN Interface Block (3ph)1/RConn3 -- F1_CB_7/LConn3
  SSN Interface Block (3ph)1/RConn6 -- F1_CB_6/LConn3
  SSN Interface Block (3ph)1/RConn4 -- F1_CB_6/LConn1
  SSN Interface Block (3ph)1/RConn5 -- F1_CB_6/LConn2
  C106/RConn2 -- 3750 kVA1/LConn2
  C106/RConn3 -- 3750 kVA1/LConn3
  C106/RConn1 -- 3750 kVA1/LConn1
  SSN Interface Block (3ph)4/RConn2 -- F1_CB_14/LConn2
  SSN Interface Block (3ph)4/RConn3 -- F1_CB_14/LConn3
  SSN Interface Block (3ph)4/RConn1 -- F1_CB_14/LConn1
  500kcmil_cable/RConn3 -- opElectricFault/LConn3
  500kcmil_cable/RConn1 -- opElectricFault/LConn1
  500kcmil_cable/RConn2 -- opElectricFault/LConn2
  500kcmil_cable1/RConn3 -- opElectricFault1/LConn3
  500kcmil_cable1/RConn1 -- opElectricFault1/LConn1
  500kcmil_cable1/RConn2 -- opElectricFault1/LConn2
  500kcmil_cable/LConn3 -- C103/RConn3 -- F1-GCB/RConn3
  500kcmil_cable/LConn2 -- C103/RConn2 -- F1-GCB/RConn2
  500kcmil_cable/LConn1 -- C103/RConn1 -- F1-GCB/RConn1
  500 kVA3/RConn3 -- Interruptible_2/LConn3
  500 kVA3/RConn2 -- Interruptible_2/LConn2
  500 kVA3/RConn1 -- Interruptible_2/LConn1
  2000 kVA4/RConn3 -- Critical_2/LConn3
  2000 kVA4/RConn1 -- Critical_2/LConn1
  2000 kVA4/RConn2 -- Critical_2/LConn2
  SSN Interface Block (3ph)4/LConn3 -- 2000 kVA5/RConn3
  SSN Interface Block (3ph)4/LConn2 -- 2000 kVA5/RConn2
  SSN Interface Block (3ph)4/LConn1 -- 2000 kVA5/RConn1
  500 kVA2/RConn3 -- Interruptible_1/LConn3
  500 kVA2/RConn2 -- Interruptible_1/LConn2
  500 kVA2/RConn1 -- Interruptible_1/LConn1
  PI-Section4/RConn3 -- F1-GCB/LConn3
  PI-Section4/RConn1 -- F1-GCB/LConn1
  PI-Section4/RConn2 -- F1-GCB/LConn2
  HWController_4MVA_DieselGenset/RConn1 -- PI-Section4/LConn1
  HWController_4MVA_DieselGenset/RConn2 -- PI-Section4/LConn2
  HWController_4MVA_DieselGenset/RConn3 -- PI-Section4/LConn3
